simulink model "psbtransfo3ph"  (Simulink 6.0)
settings: Solver=ode15s  SolverMode=SingleTasking  StartTime=0.0  StopTime=0.5  RelTol=1e-3  AbsTol=1e-2
InitFcn:
  | powericon('psbinitsys',bdroot);
libraries: powerlib2 x15, powerlib_extras x2
settings Model: Creator=patrice  LastModifiedBy=batserve  ExtModeTrigMode=oneshot  ExtModeArmWhenConnect=off  ExtModeAutoUpdateStatusClock=off
settings DataIOCC: LimitDataPoints=off  SignalLoggingName=sigsOut
settings OptimizationCC: BooleanDataType=off
settings DebuggingCC: SolverPrmCheckMsg=none  IntegerOverflowMsg=none
settings HardwareCC: TargetUnknown=on
settings RTWCC: TemplateMakefile=grt_unix.tmf

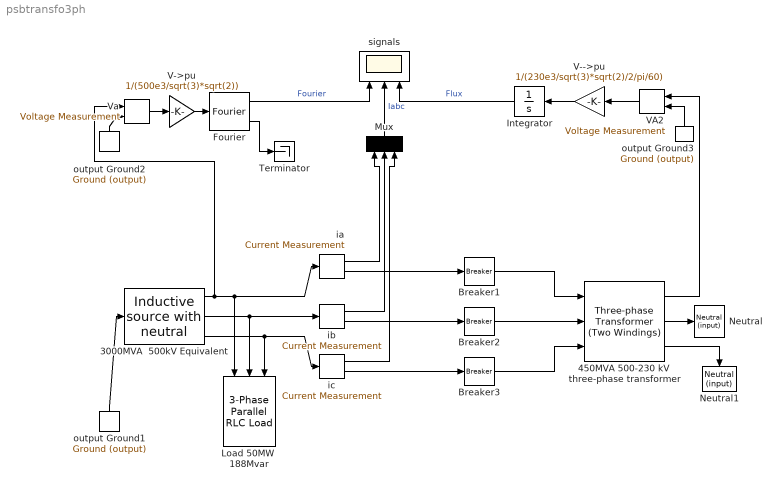
== system psbtransfo3ph ==
  3000MVA  500kV Equivalent : powerlib_extras/Three-Phase Library/Inductive source with neutral  V=500e3/sqrt(3)*sqrt(2)  Phi=0  F=60  R=5.55  L=0.221
  450MVA 500-230 kV three-phase transformer : powerlib2/Elements/Three-phase Transformer (Two Windings)  Tag=PoWeRsYsTeMbLoCk  nominal=[ 450e6 60 ]  type1=Yg  params1=[ 500e3 0.002 0.08 ]  type2=Yg  params2=[ 230e3 0.002 0.08]  ynsat=on  rmag=500  lm=500  sat="[0 0; 0.0 1.2; 1.0  1.52]"  hyst=off  matfile='hysteresis'  sif=on  phi0="[0.8  -0.4  0.4]"  initialslopes=[+1 +1 +1]  mesure=None  PSBOutputType=1111
  Breaker1 : powerlib2/Elements/Breaker  Tag=PoWeRsYsTeMbLoCk  a=1e-2  c=0  rs=100e6  cs=inf  times=.05  Ts=0  comext=off  mesure=None  PSBOutputType=1
  Breaker2 : powerlib2/Elements/Breaker  Tag=PoWeRsYsTeMbLoCk  a=1e-2  c=0  rs=100e6  cs=inf  times=.05  Ts=0  comext=off  mesure=None  PSBOutputType=1
  Breaker3 : powerlib2/Elements/Breaker  Tag=PoWeRsYsTeMbLoCk  a=1e-2  c=0  rs=100e6  cs=inf  times=.05  Ts=0  comext=off  mesure=None  PSBOutputType=1
  Fourier : powerlib_extras/Measurements/Fourier  f1=60  n=4
  Integrator : Integrator  Orientation=left  InitialCondition=0.8
  Load 50MW  188Mvar : powerlib2/Elements/3-Phase Parallel RLC Load  Orientation=down  Vpp=500e3  fn=60  P3=50e6  QL3=0  QC3=188e6
  Mux : Mux  Orientation=up  Inputs=3
  Neutral : powerlib2/Connectors/Neutral (input)  Tag=PoWeRsYsTeMbLoCk  no=991
  Neutral1 : powerlib2/Connectors/Neutral (input)  Tag=PoWeRsYsTeMbLoCk  Orientation=down  no=992
  Terminator : Terminator
  V-->pu : Gain  Orientation=left  Gain=1/(230e3/sqrt(3)*sqrt(2)/2/pi/60)  SaturateOnIntegerOverflow=on
  V->pu : Gain  Gain=1/(500e3/sqrt(3)*sqrt(2))  SaturateOnIntegerOverflow=on
  VA2 : powerlib2/Measurements/Voltage Measurement  Tag=PoWeRsYsTeMmEaSuReMeNt  Orientation=left  PhasorSimulation=off  OutputType=Magnitude  PSBOutputType=0  PSBequivalent=0
  Va : powerlib2/Measurements/Voltage Measurement  Tag=PoWeRsYsTeMmEaSuReMeNt  PhasorSimulation=off  OutputType=Magnitude  PSBOutputType=0  PSBequivalent=0
  ia : powerlib2/Measurements/Current Measurement  Tag=PoWeRsYsTeMmEaSuReMeNt  PhasorSimulation=off  OutputType=Magnitude  PSBOutputType=01  PSBequivalent=0
  ib : powerlib2/Measurements/Current Measurement  Tag=PoWeRsYsTeMmEaSuReMeNt  PhasorSimulation=off  OutputType=Magnitude  PSBOutputType=01  PSBequivalent=0
  ic : powerlib2/Measurements/Current Measurement  Tag=PoWeRsYsTeMmEaSuReMeNt  PhasorSimulation=off  OutputType=Magnitude  PSBOutputType=01  PSBequivalent=0
  output Ground1 : powerlib2/Connectors/Ground (output)  Tag=PoWeRsYsTeMbLoCk  Orientation=up  PSBOutputType=1
  output Ground2 : powerlib2/Connectors/Ground (output)  Tag=PoWeRsYsTeMbLoCk  Orientation=up  PSBOutputType=1
  output Ground3 : powerlib2/Connectors/Ground (output)  Tag=PoWeRsYsTeMbLoCk  Orientation=up  PSBOutputType=1
  signals : Scope  NumInputPorts=3
      settings: Orientation=up  TimeRange=0.2  YMin=-2000~-5~-5  YMax=3000~5~5  DataFormat=Structure
  wires:
  output Ground1/1 -> 3000MVA  500kV Equivalent/1
  3000MVA  500kV Equivalent/3 -> Load 50MW  188Mvar/3, ic/1
  3000MVA  500kV Equivalent/2 -> Load 50MW  188Mvar/2, ib/1
  ia/1 -> Mux/1
  ib/1 -> Mux/2
  ic/1 -> Mux/3
  Breaker3/1 -> 450MVA 500-230 kV three-phase transformer/3
  3000MVA  500kV Equivalent/1 -> Load 50MW  188Mvar/1, ia/1, Va/1
  450MVA 500-230 kV three-phase transformer/2 -> Neutral/1
  450MVA 500-230 kV three-phase transformer/3 -> Neutral1/1
  ia/2 -> Breaker1/1
  Breaker1/1 -> 450MVA 500-230 kV three-phase transformer/1
  Breaker2/1 -> 450MVA 500-230 kV three-phase transformer/2
  ib/2 -> Breaker2/1
  ic/2 -> Breaker3/1
  Fourier/2 -> Terminator/1
  output Ground2/1 -> Va/2
  V->pu/1 -> Fourier/1
  Va/1 -> V->pu/1
  Fourier/1 -> signals/1  "Fourier"
  Mux/1 -> signals/2  "Iabc"
  450MVA 500-230 kV three-phase transformer/1 -> VA2/1
  V-->pu/1 -> Integrator/1
  VA2/1 -> V-->pu/1
  output Ground3/1 -> VA2/2
  Integrator/1 -> signals/3  "Flux"
